simulink subsystem "Dashboard"  (R2024b)
settings: Solver=VariableStepAuto  StartTime=0.0  StopTime=10.0  RelTol=1e-3
settings Model: DataDictionary=Humidifier_Interface.sldd  EnableAccessToBaseWorkspace=off  Creator=ppatel  LastModifiedBy=ppatel

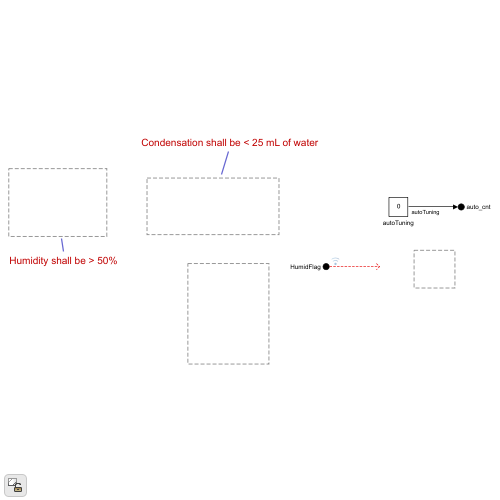
[thumbnail: Simulink's stored preview of the top-level diagram]
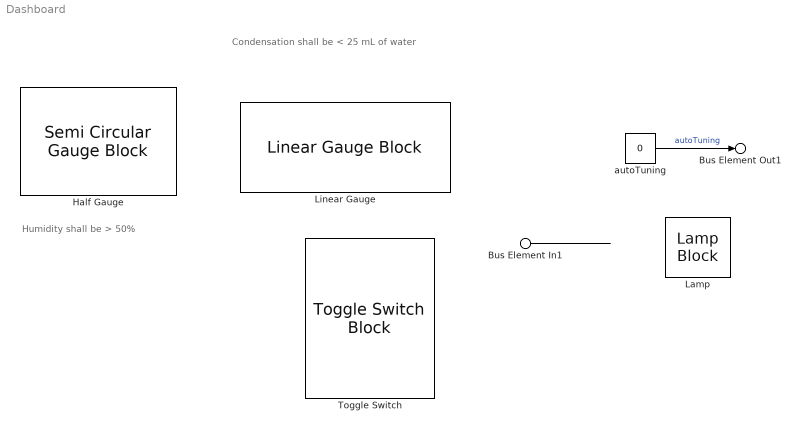
== system Dashboard ==
  note: Condensation shall be < 25 mL of water
  note: Humidity shall be > 50%
  Bus Element In1 : Inport  PortName=HumidFlag
  Half Gauge : SemiCircularGaugeBlock  TickInterval=25
  Lamp : LampBlock  LabelPosition=Hide
  Linear Gauge : LinearGaugeBlock  ScaleMax=50
  Toggle Switch : ToggleSwitchBlock
      settings: Values={{'Off', 'On'}, [0 1]}
  autoTuning : Constant  Value=0
  Bus Element Out1 : Outport  PortName=auto_cnt
  wires:
  autoTuning/1 -> Bus Element Out1/1  "autoTuning"
  Bus Element In1/1 -> ?
